simulink model "lab_10_simulink"  (R2022b)
settings: Solver=VariableStepAuto  StartTime=0.0  StopTime=50.0  RelTol=1e-3
settings Model: Creator=Ovocsiak  LastModifiedBy=huber
settings DebuggingCC: UnconnectedInputMsg=warning  UnconnectedOutputMsg=warning  UnconnectedLineMsg=warning
settings ModelReferenceCC: EnableRefExpFcnMdlSchedulingChecks=on
settings RTWCC: DLArmComputeVersion=19.05

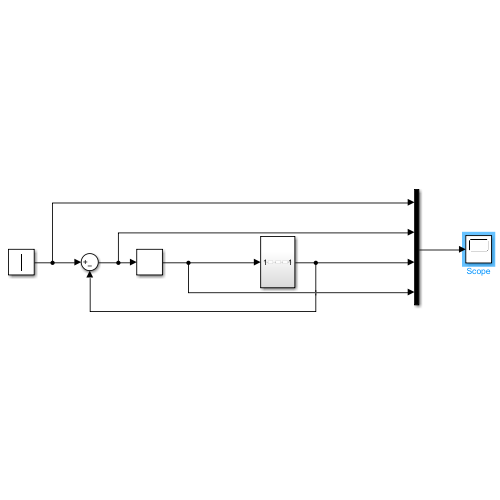
[thumbnail: Simulink's stored preview of the top-level diagram]
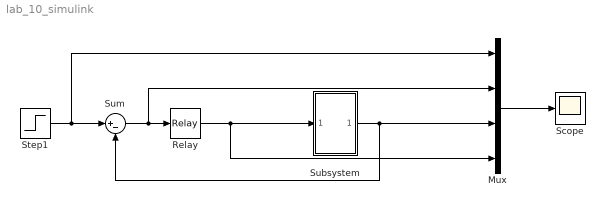
== system lab_10_simulink ==
  Mux : Mux
  Relay : Relay  OnSwitchValue=5  OffSwitchValue=-5  OnOutputValue=30
  Scope : Scope
  Step1 : Step  Time=0.1  Before=0.5  After=20  SampleTime=0
  Subsystem : Subsystem
  Sum : Sum  Inputs=|+-
  wires:
  Step1/1 -> Mux/1, Sum/1
  Mux/1 -> Scope/1
  Sum/1 -> Relay/1, Mux/2
  Relay/1 -> Subsystem/1(In1), Mux/4
  Subsystem/1(Out1) -> Mux/3, Sum/2

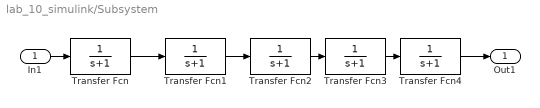
== system lab_10_simulink/Subsystem ==
  In1 : Inport
  Transfer Fcn{,1..4} (5 alike) : TransferFcn  Denominator=[1 1]
  Out1 : Outport
  wires:
  Transfer Fcn/1 -> Transfer Fcn1/1
  In1/1 -> Transfer Fcn/1
  Transfer Fcn1/1 -> Transfer Fcn2/1
  Transfer Fcn3/1 -> Transfer Fcn4/1
  Transfer Fcn2/1 -> Transfer Fcn3/1
  Transfer Fcn4/1 -> Out1/1
